simulink model "HorizontalControl"  (R2020b)
settings: Solver=VariableStepAuto  StartTime=0.0  StopTime=10.0  RelTol=1e-3
undefined symbols (not defined in the file or in its folder): A_4order, B_4order
libraries: simulink_extras x5
settings Model: Creator=JaimeParker  LastModifiedBy=JaimeParker

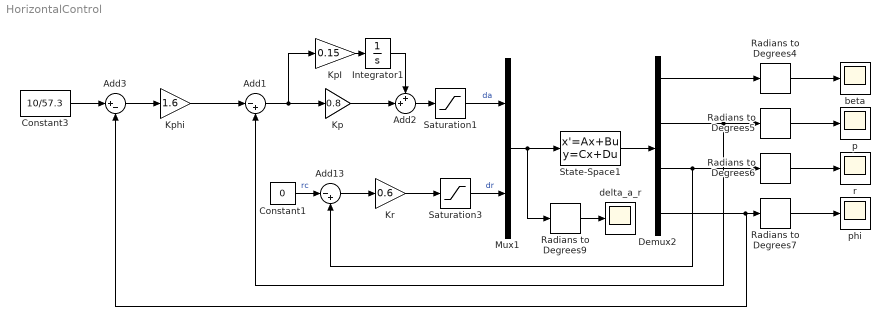
== system HorizontalControl ==
  Add1 : Sum  Inputs=|-+
  Add13 : Sum  Inputs=|-+
  Add2 : Sum  Inputs=++|
  Add3 : Sum  Inputs=|+-
  Constant1 : Constant  Value=0
  Constant3 : Constant  Value=10/57.3
  Demux2 : Demux
  Integrator1 : Integrator
  Kp : Gain  Gain=0.8
  KpI : Gain  Gain=0.15
  Kphi : Gain  Gain=1.6
  Kr : Gain  Gain=0.6
  Mux1 : Mux  Inputs=2
  Radians to Degrees{4..7,9} (5 alike) : simulink_extras/Transformations/Radians to Degrees
  Saturation1 : Saturate  UpperLimit=20/57.3  LowerLimit=-20/57.3
  Saturation3 : Saturate  UpperLimit=20/57.3  LowerLimit=-20/57.3
  State-Space1 : StateSpace  A=A_4order  B=B_4order  C=eye(4)  D=zeros(4,2)  InitialCondition=[0;0;0;0]
  beta : Scope
  delta_a_r : Scope
  p : Scope
  phi : Scope
  r : Scope
  wires:
  Demux2/3 -> Add13/2, Radians to Degrees6/1
  Kp/1 -> Add2/2
  Demux2/1 -> Radians to Degrees4/1
  Saturation1/1 -> Mux1/1  "da"
  Integrator1/1 -> Add2/1
  State-Space1/1 -> Demux2/1
  Radians to Degrees9/1 -> delta_a_r/1
  Add1/1 -> Kp/1, KpI/1
  Saturation3/1 -> Mux1/2  "dr"
  Radians to Degrees6/1 -> r/1
  Kphi/1 -> Add1/1
  KpI/1 -> Integrator1/1
  Demux2/2 -> Radians to Degrees5/1, Add1/2
  Add3/1 -> Kphi/1
  Constant3/1 -> Add3/1
  Add2/1 -> Saturation1/1
  Radians to Degrees5/1 -> p/1
  Constant1/1 -> Add13/1  "rc"
  Demux2/4 -> Add3/2, Radians to Degrees7/1
  Add13/1 -> Kr/1
  Radians to Degrees7/1 -> phi/1
  Mux1/1 -> Radians to Degrees9/1, State-Space1/1
  Radians to Degrees4/1 -> beta/1
  Kr/1 -> Saturation3/1
